simulink model "JGVD_Mixing_Tank_PID"  (R2022a)
settings: Solver=VariableStepAuto  StartTime=0.0  StopTime=200  RelTol=1e-3
values from neighbouring files (symbols this model uses):
  alphaD = 0.2    [JGVD_Mixing_Tank_Parameters.m]    (also in JGVD_Non_Isothermal_CSTR_Parameters.m)
  kC_PID = 1/(kP*kV)    [JGVD_Mixing_Tank_Parameters.m]    (also in JGVD_Non_Isothermal_CSTR_Parameters.m = 1/(kP*kV*100))
  kD = dv.deltaY/dv.deltaX    [JGVD_Mixing_Tank_Parameters.m]    (also in JGVD_Non_Isothermal_CSTR_Parameters.m)
  kP = cv.deltaY/cv.deltaX    [JGVD_Mixing_Tank_Parameters.m]    (also in JGVD_Non_Isothermal_CSTR_Parameters.m)
  tauD = 1.5*(dv.t_63-dv.t_28)    [JGVD_Mixing_Tank_Parameters.m]    (also in JGVD_Non_Isothermal_CSTR_Parameters.m)
  tauP = 1.5*(cv.t_63-cv.t_28)    [JGVD_Mixing_Tank_Parameters.m]    (also in JGVD_Non_Isothermal_CSTR_Parameters.m)
  TD_PID = 0.05*(thetaP+tauP)    [JGVD_Mixing_Tank_Parameters.m]    (also in JGVD_Non_Isothermal_CSTR_Parameters.m)
  thetaD = dv.t_63-tauD    [JGVD_Mixing_Tank_Parameters.m]    (also in JGVD_Non_Isothermal_CSTR_Parameters.m)
  thetaP = cv.t_63-tauP    [JGVD_Mixing_Tank_Parameters.m]    (also in JGVD_Non_Isothermal_CSTR_Parameters.m)
  TI_PID = 0.82*(thetaP+tauP)    [JGVD_Mixing_Tank_Parameters.m]    (also in JGVD_Non_Isothermal_CSTR_Parameters.m)
  xA = ((p.F1 + p.F2)*xA_0)/(p.F1 + p.F2)    [JGVD_Mixing_Tank_Parameters.m]
undefined symbols (not defined in the file or in its folder): p
settings Model: Creator=georg  LastModifiedBy=georg
settings SolverCC: ZeroCrossAlgorithm=Adaptive
settings DebuggingCC: IgnoredZcDiagnostic=none

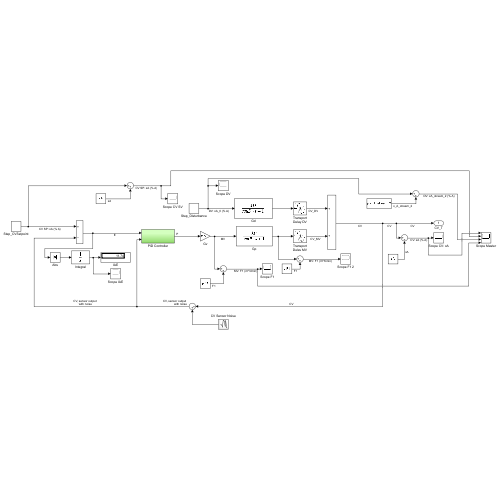
[thumbnail: Simulink's stored preview of the top-level diagram]
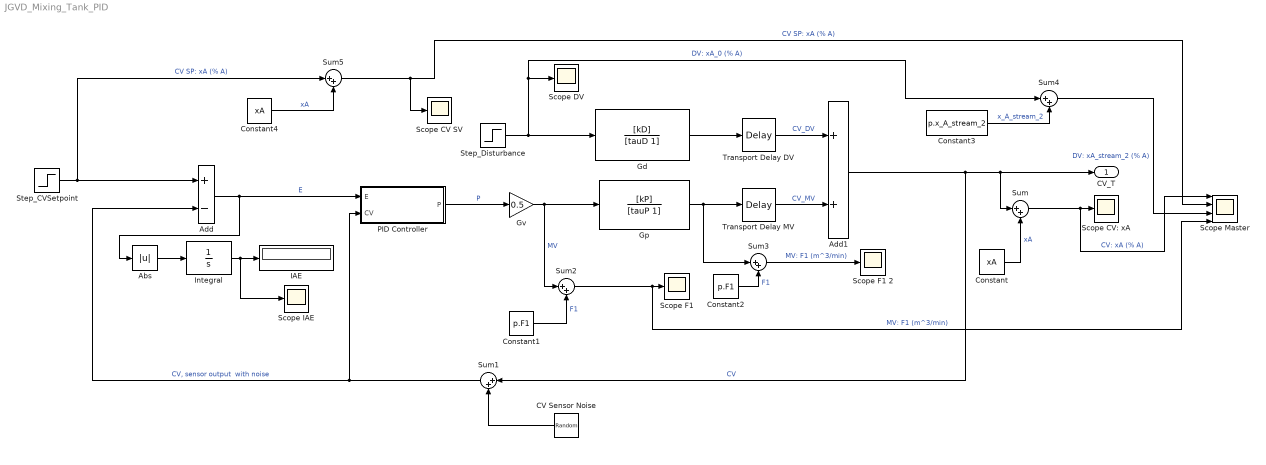
== system JGVD_Mixing_Tank_PID ==
  "Abs " : Abs  SaturateOnIntegerOverflow=off
  Add : Sum  Inputs=+-
  Add1 : Sum
  CV Sensor Noise : RandomNumber  Variance=5*10^-4  Seed=4  SampleTime=0.2
  Constant : Constant  Value=xA
  Constant1 : Constant  Value=p.F1
  Constant2 : Constant  Value=p.F1
  Constant3 : Constant  Value=p.x_A_stream_2
  Constant4 : Constant  Value=xA
  Gd : TransferFcn  Numerator=[kD]  Denominator=[tauD 1]
  Gp : TransferFcn  Numerator=[kP]  Denominator=[tauP 1]
  Gv : Gain  Gain=0.5
  IAE : Display
  Integral : Integrator
  PID Controller : Subsystem
  "Scope CV SV " : Scope
  Scope CV: xA : Scope
  Scope DV : Scope
  Scope F1 : Scope
  Scope F1 2 : Scope
  Scope IAE : Scope
  Scope Master : Scope  NumInputPorts=4
  Step_CVSetpoint : Step  Time=20  After=xA*0.05  SampleTime=0
  Step_Disturbance : Step  Time=100  After=p.x_A_stream_2*2  SampleTime=0
  Sum{,1..5} (6 alike) : Sum  Inputs=|++
  Transport Delay DV : TransportDelay  DelayTime=thetaD
  Transport Delay MV : TransportDelay  DelayTime=thetaP
  CV_T : Outport  VectorParamsAs1DForOutWhenUnconnected=off
  wires:
  Transport Delay DV/1 -> Add1/1  "CV_DV"
  Constant/1 -> Sum/2  "xA"
  Integral/1 -> Scope IAE/1, IAE/1
  "Abs "/1 -> Integral/1
  Transport Delay MV/1 -> Add1/2  "CV_MV"
  Step_CVSetpoint/1 -> Sum5/1, Add/1  "CV SP: xA (% A)"
  Add/1 -> "Abs "/1, PID Controller/1(E)  "E"
  Gp/1 -> Sum3/1, Transport Delay MV/1
  Add1/1 -> Sum/1, CV_T/1, Sum1/1  "CV"
  Gv/1 -> Sum2/1, Gp/1  "MV"
  Gd/1 -> Transport Delay DV/1
  Step_Disturbance/1 -> Sum4/1, Scope DV/1, Gd/1  "DV: xA_0 (% A)"
  Sum/1 -> Scope Master/1, Scope CV: xA/1  "CV: xA (% A)"
  PID Controller/1(P) -> Gv/1  "P"
  CV Sensor Noise/1 -> Sum1/2
  Sum1/1 -> Add/2, PID Controller/2(CV)  "CV, sensor output  with noise"
  Sum2/1 -> Scope Master/4, Scope F1/1  "MV: F1 (m^3/min)"
  Constant1/1 -> Sum2/2  "F1"
  Constant2/1 -> Sum3/2  "F1"
  Sum3/1 -> Scope F1 2/1  "MV: F1 (m^3/min)"
  Sum4/1 -> Scope Master/3  "DV: xA_stream_2 (% A)"
  Constant3/1 -> Sum4/2  "x_A_stream_2"
  Constant4/1 -> Sum5/2  "xA"
  Sum5/1 -> "Scope CV SV "/1, Scope Master/2  "CV SP: xA (% A)"

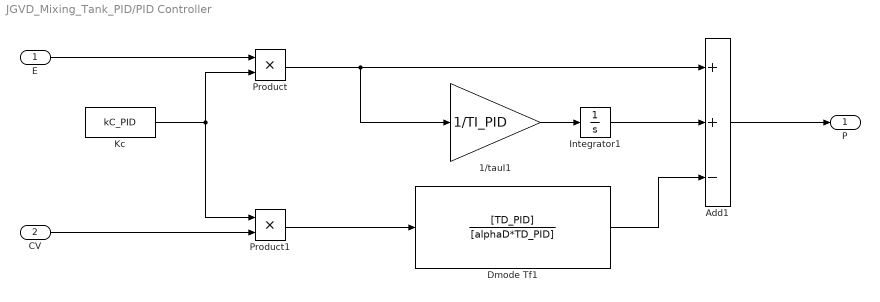
== system JGVD_Mixing_Tank_PID/PID Controller ==
  E : Inport
  CV : Inport  Port=2
  1/tauI1 : Gain  Gain=1/TI_PID
  Add1 : Sum  Inputs=++-
  Dmode Tf1 : TransferFcn  Numerator=[TD_PID]  Denominator=[alphaD*TD_PID]
  Integrator1 : Integrator
  Kc : Constant  Value=kC_PID
  Product : Product
  Product1 : Product
  P : Outport  VectorParamsAs1DForOutWhenUnconnected=off
  wires:
  CV/1 -> Product1/2
  Product1/1 -> Dmode Tf1/1
  1/tauI1/1 -> Integrator1/1
  Product/1 -> 1/tauI1/1, Add1/1
  Add1/1 -> P/1
  Integrator1/1 -> Add1/2
  Dmode Tf1/1 -> Add1/3
  E/1 -> Product/1
  Kc/1 -> Product/2, Product1/1
